simulink model "P2_Ex9a"  (R2018a)
settings: Solver=VariableStepAuto  StartTime=0.0  StopTime=10.0  RelTol=1e-3
values from neighbouring files (symbols this model uses):
  K0 = 0.82/0.017    (= 48.2352941176)    [Ex9_preload.m]
  Kp = 1    [Ex9_preload.m]
  Kt = 0.017    [Ex9_preload.m]
  tau0 = 0.26    [Ex9_preload.m]
  Ts = 0.01    [Ex9_preload.m]
settings Model: Creator=Eneko Lerma  LastModifiedBy=Eneko Lerma

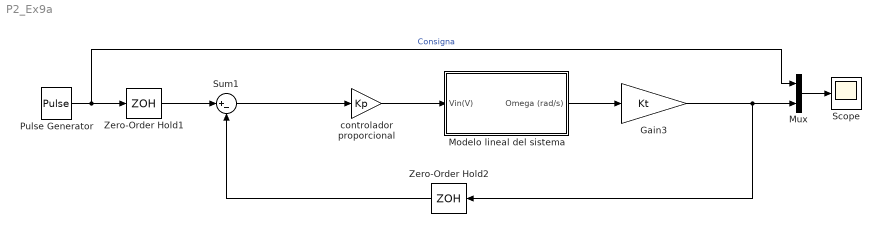
== system P2_Ex9a ==
  Gain3 : Gain  Gain=Kt
  Modelo lineal del sistema : Subsystem
  Mux : Mux  Inputs=2
  Pulse Generator : DiscretePulseGenerator  PulseType=Time based  Period=5  PulseWidth=50
  Scope : Scope
  Sum1 : Sum  Inputs=|+-
  Zero-Order Hold1 : ZeroOrderHold  SampleTime=Ts
  Zero-Order Hold2 : ZeroOrderHold  SampleTime=Ts
  controlador proporcional : Gain  Gain=Kp
  wires:
  Sum1/1 -> controlador proporcional/1
  Pulse Generator/1 -> Mux/1, Zero-Order Hold1/1  "Consigna"
  Gain3/1 -> Zero-Order Hold2/1, Mux/2
  Mux/1 -> Scope/1
  controlador proporcional/1 -> Modelo lineal del sistema/1(Vin(V))
  Modelo lineal del sistema/1(Omega (rad/s)) -> Gain3/1
  Zero-Order Hold1/1 -> Sum1/1
  Zero-Order Hold2/1 -> Sum1/2

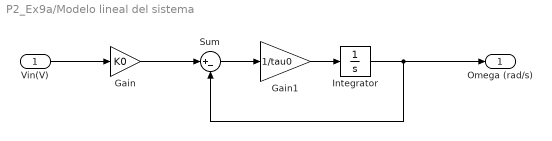
== system P2_Ex9a/Modelo lineal del sistema ==
  Vin(V) : Inport
  Gain : Gain  Gain=K0
  Gain1 : Gain  Gain=1/tau0
  Integrator : Integrator
  Sum : Sum  Inputs=|+-
  Omega (rad/s) : Outport
  wires:
  Integrator/1 -> Omega (rad/s)/1, Sum/2
  Sum/1 -> Gain1/1
  Vin(V)/1 -> Gain/1
  Gain1/1 -> Integrator/1
  Gain/1 -> Sum/1
